simulink model "Test1"  (R2017b)
settings: Solver=VariableStepAuto  StartTime=0.0  StopTime=10.0  RelTol=1e-3
undefined symbols (not defined in the file): br, bt, g, l, m, M
settings Model: Creator=Benjamin Nicolas  LastModifiedBy=Benjamin Nicolas

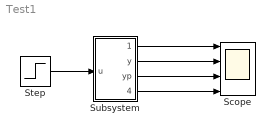
== system Test1 ==
  Scope : Scope  NumInputPorts=4
  Step : Step  SampleTime=0
  Subsystem : Subsystem
  wires:
  Subsystem/1(theta) -> Scope/1
  Subsystem/2(y) -> Scope/2
  Subsystem/3(yp) -> Scope/3
  Subsystem/4(thetap) -> Scope/4
  Step/1 -> Subsystem/1("u ")

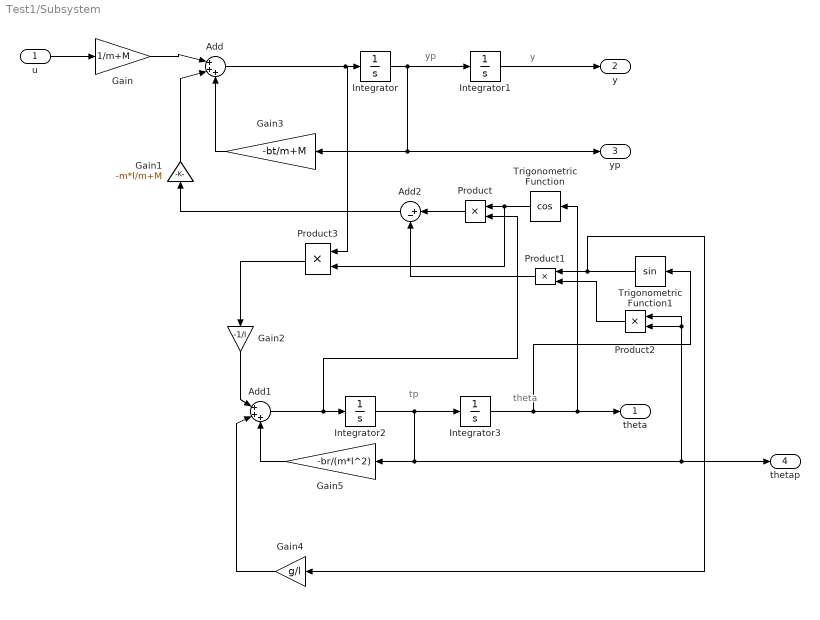
== system Test1/Subsystem ==
  note: y
  note: theta
  note: tp
  note: yp
  "u " : Inport
  Add : Sum  Inputs=|+++
  Add1 : Sum  Inputs=|+++
  Add2 : Sum  Inputs=|+-
  Gain : Gain  Gain=1/m+M
  Gain1 : Gain  Gain=-m*l/m+M
  Gain2 : Gain  Gain=-1/l
  Gain3 : Gain  Gain=-bt/m+M
  Gain4 : Gain  Gain=g/l
  Gain5 : Gain  Gain=-br/(m*l^2)
  Integrator : Integrator
  Integrator1 : Integrator
  Integrator2 : Integrator
  Integrator3 : Integrator  InitialCondition=0.1
  Product{,1..3} (4 alike) : Product
  Trigonometric Function : Trigonometry  Operator=cos
  Trigonometric Function1 : Trigonometry
  theta : Outport
  y : Outport  Port=2
  yp : Outport  Port=3
  thetap : Outport  Port=4
  wires:
  Gain4/1 -> Add1/2
  Gain3/1 -> Add/3
  Product3/1 -> Gain2/1
  Trigonometric Function1/1 -> Gain4/1, Product1/1
  Product/1 -> Add2/1
  Gain2/1 -> Add1/1
  Gain1/1 -> Add/2
  Add1/1 -> Product/2, Integrator2/1
  Gain/1 -> Add/1
  Add2/1 -> Gain1/1
  Integrator3/1 -> Trigonometric Function1/1, theta/1, Trigonometric Function/1
  Product1/1 -> Add2/2
  "u "/1 -> Gain/1
  Product2/1 -> Product1/2
  Gain5/1 -> Add1/3
  Trigonometric Function/1 -> Product3/2, Product/1
  Integrator2/1 -> Integrator3/1, Product2/1, Product2/2, thetap/1, Gain5/1
  Add/1 -> Integrator/1, Product3/1
  Integrator/1 -> yp/1, Gain3/1, Integrator1/1
  Integrator1/1 -> y/1
